simulink model "se"  (R2018a)
settings: Solver=VariableStepAuto  StartTime=0.0  StopTime=3e-5  RelTol=1e-3
undefined symbols (not defined in the file or in its folder): Ae, Be, C, Ce, De, L, R1, R2
settings Model: Creator=carma  LastModifiedBy=carma

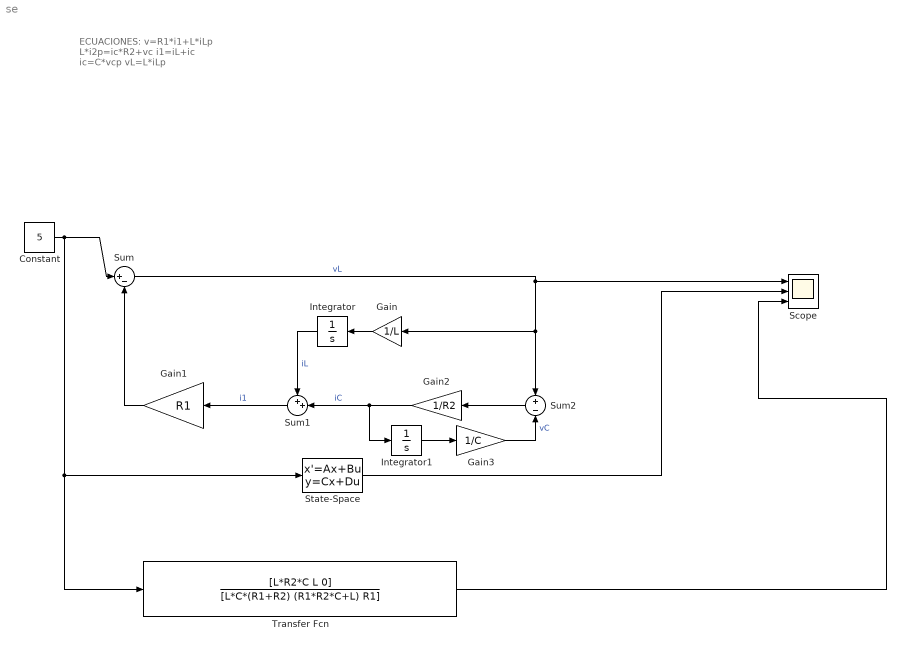
== system se ==
  note: ECUACIONES:
      | v=R1*i1+L*iLp
      | L*i2p=ic*R2+vc
      | i1=iL+ic
      | ic=C*vcp
      | vL=L*iLp
  Constant : Constant  Value=5
  Gain : Gain  Gain=1/L
  Gain1 : Gain  Gain=R1
  Gain2 : Gain  Gain=1/R2
  Gain3 : Gain  Gain=1/C
  Integrator : Integrator
  Integrator1 : Integrator
  Scope : Scope  NumInputPorts=3
  State-Space : StateSpace  A=Ae  B=Be  C=Ce  D=De  InitialCondition=0
  Sum : Sum  Inputs=|+-
  Sum1 : Sum  Inputs=++|
  Sum2 : Sum  Inputs=+-
  Transfer Fcn : TransferFcn  Numerator=[L*R2*C L 0]  Denominator=[L*C*(R1+R2) (R1*R2*C+L) R1]
  wires:
  Sum/1 -> Sum2/1, Gain/1, Scope/1  "vL"
  Sum1/1 -> Gain1/1  "i1"
  Gain1/1 -> Sum/2
  Constant/1 -> Transfer Fcn/1, State-Space/1, Sum/1
  State-Space/1 -> Scope/2
  Transfer Fcn/1 -> Scope/3
  Gain/1 -> Integrator/1
  Integrator/1 -> Sum1/1  "iL"
  Sum2/1 -> Gain2/1
  Integrator1/1 -> Gain3/1
  Gain2/1 -> Integrator1/1, Sum1/2  "iC"
  Gain3/1 -> Sum2/2  "vC"
